simulink subsystem "ANDI"  (R2019b)
settings: Solver=VariableStepAuto  StartTime=0.0  StopTime=10.0  RelTol=1e-3
settings Model: Creator=mauro  LastModifiedBy=mauro

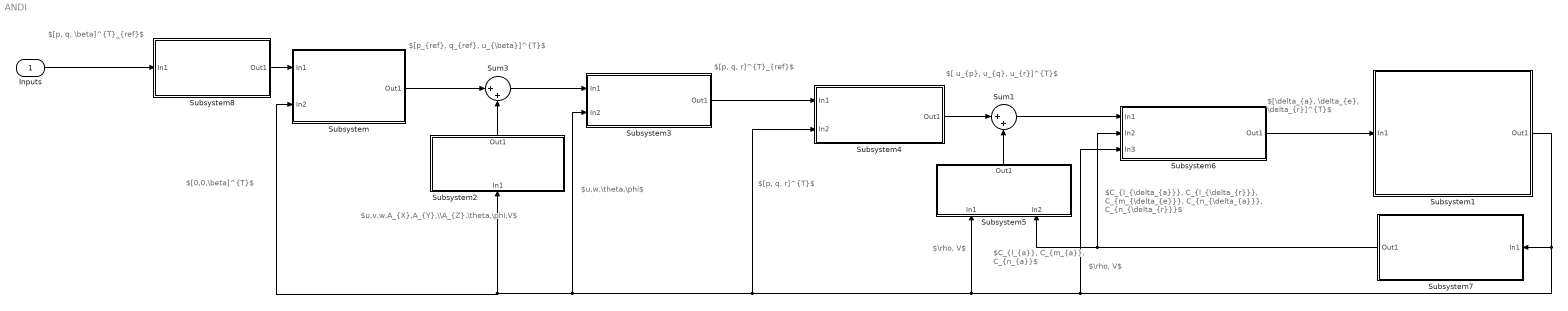
== system ANDI ==
  note: $[p, q, r]^{T}_{ref}$
  note: $[p_{ref}, q_{ref}, \nu_{\beta}]^{T}$
  note: $[\nu_{p}, \nu_{q}, \nu_{r}]^{T}$
  note: $[\delta_{a}, \delta_{e}, \delta_{r}]^{T}$
  note: $C_{l_{\delta_{a}}}, C_{l_{\delta_{r}}}, C_{m_{\delta_{e}}}, C_{n_{\delta_{a}}}, C_{n_{\delta_{r}}}$
  note: $C_{l_{a}}, C_{m_{a}}, C_{n_{a}}$
  note: $\rho, V$
  note: $\rho, V$
  note: $[0,0,\beta]^{T}$
  note: $[p, q, r]^{T}$
  note: $u,v,w,A_{X},A_{Y},\\A_{Z},\theta,\phi,V$
  note: $u,w,\theta,\phi$
  note: $[p, q, \beta]^{T}_{ref}$
  Inputs : Inport
  Subsystem : Subsystem
      mask Display: image("C:\Users\mauro\OneDrive\AE Master - TU Delft\Nonlinear and Adaptive Flight Control (AE4311)\AE4311_FTFCAssignment\cessna_model\controller_fig\lc_2.png")
  Subsystem1 : Subsystem
      mask Display: image("C:\Users\mauro\OneDrive\AE Master - TU Delft\Nonlinear and Adaptive Flight Control (AE4311)\AE4311_FTFCAssignment\cessna_model\controller_fig\ac.jpg")
  Subsystem2 : Subsystem
      mask Display: image("C:\Users\mauro\OneDrive\AE Master - TU Delft\Nonlinear and Adaptive Flight Control (AE4311)\AE4311_FTFCAssignment\cessna_model\controller_fig\a_kyn.png")
  Subsystem3 : Subsystem
      mask Display: image("C:\Users\mauro\OneDrive\AE Master - TU Delft\Nonlinear and Adaptive Flight Control (AE4311)\AE4311_FTFCAssignment\cessna_model\controller_fig\b_kyn.png")
  Subsystem4 : Subsystem
      mask Display: image("C:\Users\mauro\OneDrive\AE Master - TU Delft\Nonlinear and Adaptive Flight Control (AE4311)\AE4311_FTFCAssignment\cessna_model\controller_fig\lc_1.png")
  Subsystem5 : Subsystem
      mask Display: image("C:\Users\mauro\OneDrive\AE Master - TU Delft\Nonlinear and Adaptive Flight Control (AE4311)\AE4311_FTFCAssignment\cessna_model\controller_fig\a_dyn.png")
  Subsystem6 : Subsystem
      mask Display: image("C:\Users\mauro\OneDrive\AE Master - TU Delft\Nonlinear and Adaptive Flight Control (AE4311)\AE4311_FTFCAssignment\cessna_model\controller_fig\b_dyn.png")
  Subsystem7 : Subsystem
      mask Display: image("C:\Users\mauro\OneDrive\AE Master - TU Delft\Nonlinear and Adaptive Flight Control (AE4311)\AE4311_FTFCAssignment\cessna_model\controller_fig\ami.png")
  Subsystem8 : Subsystem
      mask Display: image("C:\Users\mauro\OneDrive\AE Master - TU Delft\Nonlinear and Adaptive Flight Control (AE4311)\AE4311_FTFCAssignment\cessna_model\controller_fig\lpf.png")
  Sum1 : Sum  Inputs=|++
  Sum3 : Sum  Inputs=|++
  wires:
  Inputs/1 -> Subsystem8/1(In1)
  Subsystem1/1(Out1) -> Subsystem/2(In2), Subsystem2/1(In1), Subsystem3/2(In2), Subsystem4/2(In2), Subsystem5/1(In1), Subsystem6/3(In3), Subsystem7/1(In1)
  Subsystem/1(Out1) -> Sum3/1
  Subsystem2/1(Out1) -> Sum3/2
  Sum3/1 -> Subsystem3/1(In1)
  Subsystem3/1(Out1) -> Subsystem4/1(In1)
  Subsystem4/1(Out1) -> Sum1/1
  Subsystem5/1(Out1) -> Sum1/2
  Sum1/1 -> Subsystem6/1(In1)
  Subsystem6/1(Out1) -> Subsystem1/1(In1)
  Subsystem7/1(Out1) -> Subsystem6/2(In2), Subsystem5/2(In2)
  Subsystem8/1(Out1) -> Subsystem/1(In1)

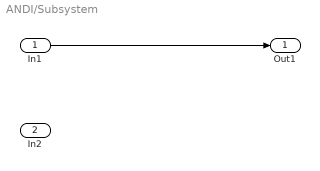
== system ANDI/Subsystem ==
  In1 : Inport
  In2 : Inport  Port=2
  Out1 : Outport
  wires:
  In1/1 -> Out1/1

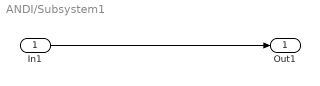
== system ANDI/Subsystem1 ==
  In1 : Inport
  Out1 : Outport
  wires:
  In1/1 -> Out1/1

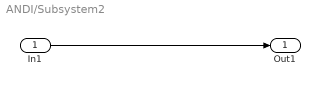
== system ANDI/Subsystem2 ==
  In1 : Inport
  Out1 : Outport
  wires:
  In1/1 -> Out1/1

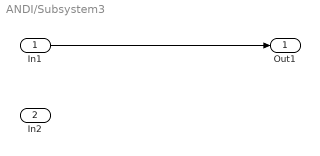
== system ANDI/Subsystem3 ==
  In1 : Inport
  In2 : Inport  Port=2
  Out1 : Outport
  wires:
  In1/1 -> Out1/1

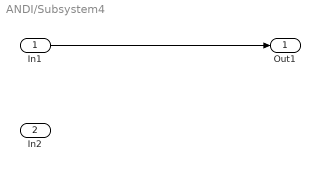
== system ANDI/Subsystem4 ==
  In1 : Inport
  In2 : Inport  Port=2
  Out1 : Outport
  wires:
  In1/1 -> Out1/1

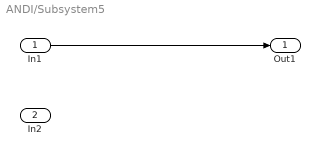
== system ANDI/Subsystem5 ==
  In1 : Inport
  In2 : Inport  Port=2
  Out1 : Outport
  wires:
  In1/1 -> Out1/1

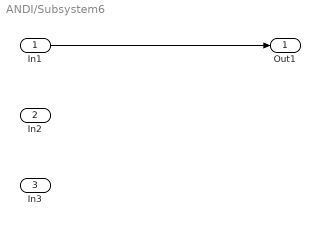
== system ANDI/Subsystem6 ==
  In1 : Inport
  In2 : Inport  Port=2
  In3 : Inport  Port=3
  Out1 : Outport
  wires:
  In1/1 -> Out1/1

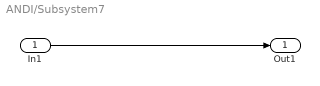
== system ANDI/Subsystem7 ==
  In1 : Inport
  Out1 : Outport
  wires:
  In1/1 -> Out1/1

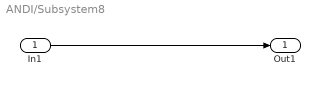
== system ANDI/Subsystem8 ==
  In1 : Inport
  Out1 : Outport
  wires:
  In1/1 -> Out1/1
